simulink model "PD"  (R2022b)
settings: Solver=VariableStepAuto  StartTime=0.0  StopTime=10.0  RelTol=1e-3
libraries: simulink x1
settings Model: Creator=Vikhyath  LastModifiedBy=Vikhyath

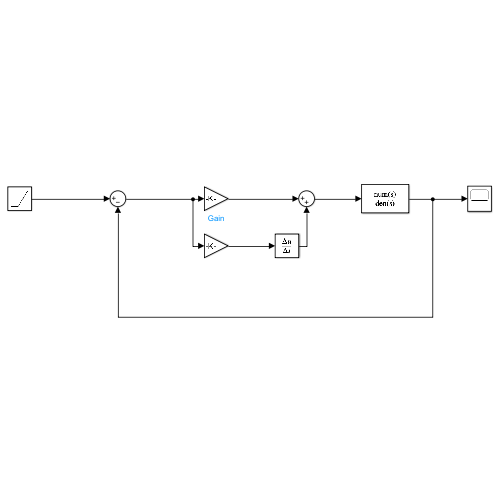
[thumbnail: Simulink's stored preview of the top-level diagram]
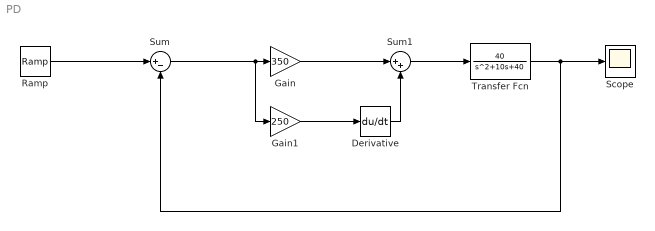
== system PD ==
  Derivative : Derivative
  Gain : Gain  Gain=350
  Gain1 : Gain  Gain=250
  Ramp : simulink/Sources/Ramp  slope=0  start=0  InitialOutput=0
  Scope : Scope
  Sum : Sum  Inputs=|+-
  Sum1 : Sum  Inputs=|++
  Transfer Fcn : TransferFcn  Numerator=[40]  Denominator=[1 10 40]
  wires:
  Ramp/1 -> Sum/1
  Sum/1 -> Gain1/1, Gain/1
  Gain/1 -> Sum1/1
  Sum1/1 -> Transfer Fcn/1
  Gain1/1 -> Derivative/1
  Derivative/1 -> Sum1/2
  Transfer Fcn/1 -> Sum/2, Scope/1
